simulink model "laneselect"  (R2016a)
settings: Solver=VariableStepAuto  StartTime=0.0  StopTime=10.0  RelTol=1e-3
settings Model: Creator=NBGD  LastModifiedBy=NBGD

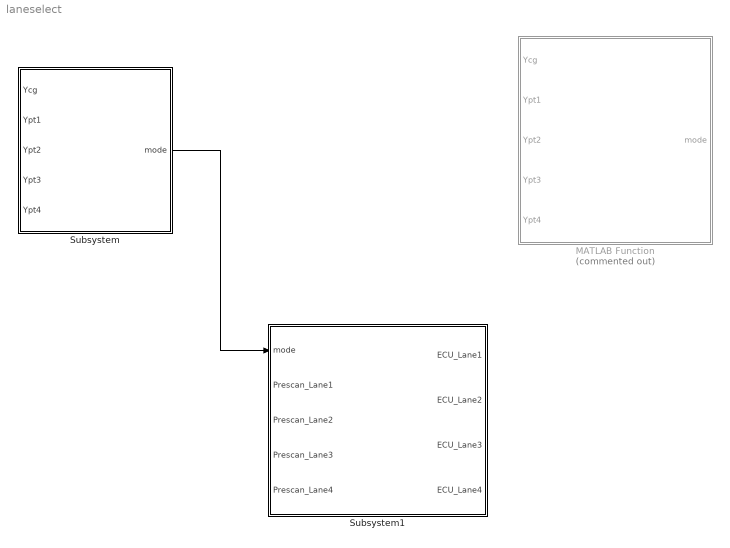
== system laneselect ==
  MATLAB Function : MATLAB Function  Commented=on  TreatAsAtomicUnit=on
  Subsystem : Subsystem
  Subsystem1 : Subsystem
  wires:
  Subsystem/1(mode) -> Subsystem1/1(mode)

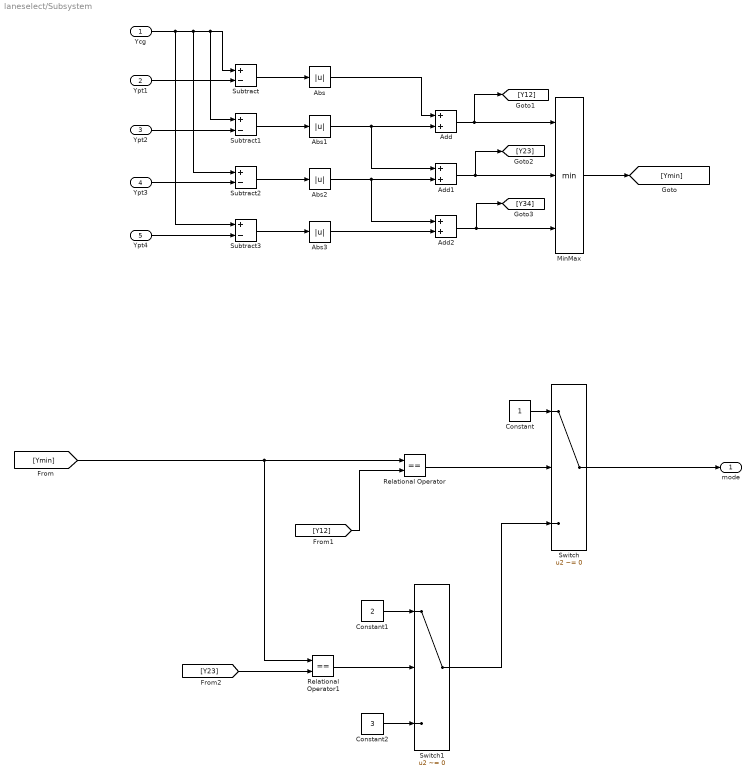
== system laneselect/Subsystem ==
  Ycg : Inport
  Ypt1 : Inport  Port=2
  Ypt2 : Inport  Port=3
  Ypt3 : Inport  Port=4
  Ypt4 : Inport  Port=5
  Abs{,1..3} (4 alike) : Abs
  Add : Sum
  Add1 : Sum
  Add2 : Sum
  Constant : Constant
  Constant1 : Constant  Value=2
  Constant2 : Constant  Value=3
  MinMax : MinMax  Inputs=3
  Relational Operator : RelationalOperator  Operator===  OutDataTypeStr=boolean
  Relational Operator1 : RelationalOperator  Operator===  OutDataTypeStr=boolean
  Subtract{,1..3} (4 alike) : Sum  Inputs=+-
  Switch : Switch  Criteria=u2 ~= 0
  Switch1 : Switch  Criteria=u2 ~= 0
  mode : Outport
  wires:
  Ycg/1 -> Subtract3/1, Subtract2/1, Subtract1/1, Subtract/1
  Abs/1 -> Add/1
  Ypt1/1 -> Subtract/2
  Subtract/1 -> Abs/1
  Ypt2/1 -> Subtract1/2
  Ypt3/1 -> Subtract2/2
  Ypt4/1 -> Subtract3/2
  Subtract2/1 -> Abs2/1
  Subtract3/1 -> Abs3/1
  Subtract1/1 -> Abs1/1
  Abs1/1 -> Add1/1, Add/2
  Abs2/1 -> Add2/1, Add1/2
  Abs3/1 -> Add2/2
  Add1/1 -> [Y23], MinMax/2
  Add/1 -> [Y12], MinMax/1
  Add2/1 -> [Y34], MinMax/3
  MinMax/1 -> [Ymin]
  Constant/1 -> Switch/1
  [Ymin] -> Relational Operator1/1, Relational Operator/1
  [Y12] -> Relational Operator/2
  Relational Operator/1 -> Switch/2
  Switch1/1 -> Switch/3
  Constant1/1 -> Switch1/1
  Relational Operator1/1 -> Switch1/2
  [Y23] -> Relational Operator1/2
  Constant2/1 -> Switch1/3
  Switch/1 -> mode/1

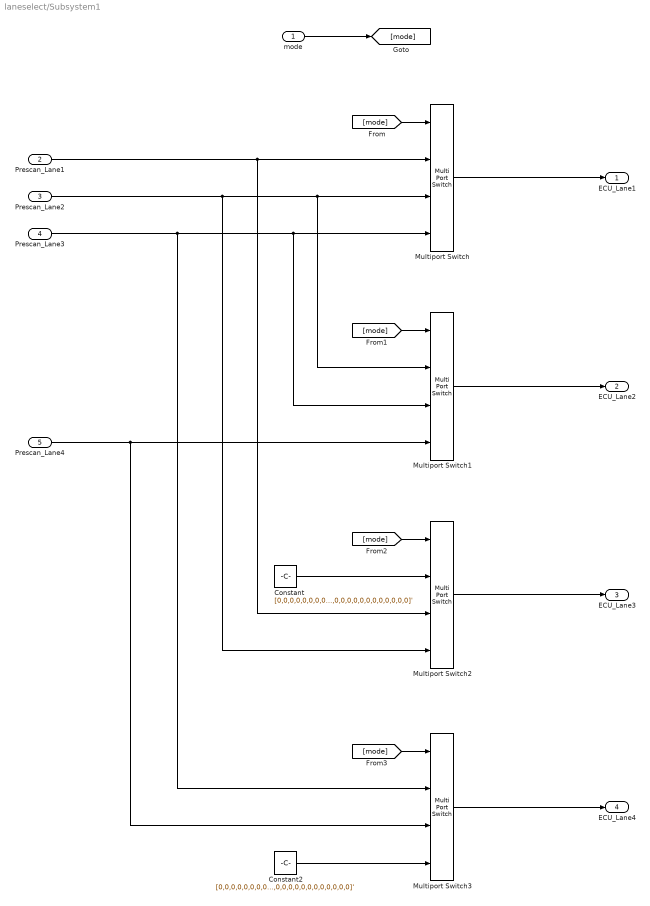
== system laneselect/Subsystem1 ==
  mode : Inport
  Prescan_Lane1 : Inport  Port=2
  Prescan_Lane2 : Inport  Port=3
  Prescan_Lane3 : Inport  Port=4
  Prescan_Lane4 : Inport  Port=5
  Constant : Constant  Value=[0,0,0,0,0,0,0,0,0,0,0,0,0,0,0,0,0,0,0,0]'
  Constant2 : Constant  Value=[0,0,0,0,0,0,0,0,0,0,0,0,0,0,0,0,0,0,0,0]'
  Multiport Switch{,1..3} (4 alike) : MultiPortSwitch
  ECU_Lane1 : Outport
  ECU_Lane2 : Outport  Port=2
  ECU_Lane3 : Outport  Port=3
  ECU_Lane4 : Outport  Port=4
  wires:
  [mode] -> Multiport Switch/1
  Prescan_Lane1/1 -> Multiport Switch2/3, Multiport Switch/2
  Multiport Switch/1 -> ECU_Lane1/1
  [mode] -> Multiport Switch1/1
  Multiport Switch1/1 -> ECU_Lane2/1
  Prescan_Lane4/1 -> Multiport Switch3/3, Multiport Switch1/4
  mode/1 -> [mode]
  [mode] -> Multiport Switch2/1
  Constant/1 -> Multiport Switch2/2
  Multiport Switch2/1 -> ECU_Lane3/1
  Prescan_Lane2/1 -> Multiport Switch2/4, Multiport Switch1/2, Multiport Switch/3
  [mode] -> Multiport Switch3/1
  Prescan_Lane3/1 -> Multiport Switch3/2, Multiport Switch1/3, Multiport Switch/4
  Multiport Switch3/1 -> ECU_Lane4/1
  Constant2/1 -> Multiport Switch3/4

== matlab function laneselect/MATLAB Function ==
  data: Ycg input; mode output; Ypt1 input; Ypt2 input; Ypt3 input; Ypt4 input
function mode= fcn(Ycg,Ypt1,Ypt2,Ypt3,Ypt4)
%#codegen
temp1 = abs(Ypt1-Ycg)+abs(Ypt2-Ycg);
temp2 = abs(Ypt2-Ycg)+abs(Ypt3-Ycg);
temp3 = abs(Ypt3-Ycg)+abs(Ypt4-Ycg);
temp  = min(temp1,temp2,temp3);
if temp==temp1
    i=1;
elseif temp==temp2
    i=2;
else
    i=3;
end
mode = i;
